simulink model "undirect_graph_disturbance_first_order_switch"  (R2020a)
settings: Solver=FixedStepAuto  StartTime=0.0  StopTime=10.0  FixedStep=0.0001  RelTol=1e-3
libraries: simulink x10, fod x1
settings Model: Creator=WangQipeng  LastModifiedBy=WangQipeng

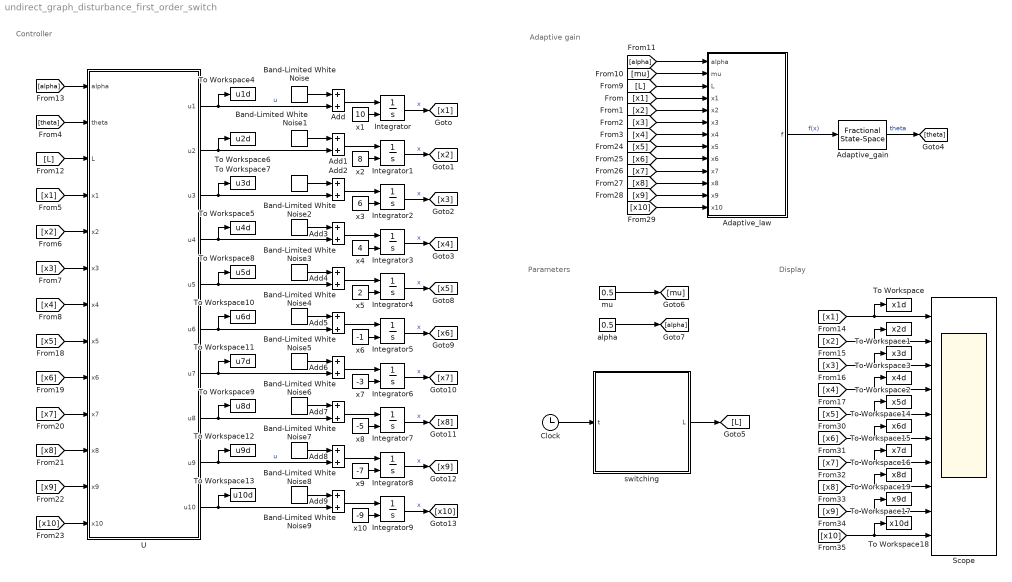
== system undirect_graph_disturbance_first_order_switch ==
  note: Controller
  note: Adaptive gain
  note: Display
  note: Parameters
  Adaptive_gain : fod/Fractional State-Space  A=0  B=1  C=1  D=0  q=0.5  iniOff=[0]  freqRange=[0.0001 10000]  approxNum=5  useRef=off  mask(FOSS){}
      settings: SourceProductName=FOMCON Toolbox
      mask Display: disp(['D^\beta \theta=f(x)'], 'TeXMode', 'On');
  Adaptive_law : MATLAB Function  TreatAsAtomicUnit=on
  Add{,1..9} (10 alike) : Sum
  Band-Limited White Noise : simulink/Sources/Band-Limited White Noise  Cov=[0.01]  Ts=0.01  seed=[23341]
  Band-Limited White Noise1 : simulink/Sources/Band-Limited White Noise  Cov=[0.01]  Ts=0.01  seed=[22141]
  Band-Limited White Noise2 : simulink/Sources/Band-Limited White Noise  Cov=[0.01]  Ts=0.01  seed=[27541]
  Band-Limited White Noise3 : simulink/Sources/Band-Limited White Noise  Cov=[0.01]  Ts=0.01  seed=[23841]
  Band-Limited White Noise4 : simulink/Sources/Band-Limited White Noise  Cov=[0.01]  Ts=0.01  seed=[25341]
  Band-Limited White Noise5 : simulink/Sources/Band-Limited White Noise  Cov=[0.01]  Ts=0.01  seed=[23261]
  Band-Limited White Noise6 : simulink/Sources/Band-Limited White Noise  Cov=[0.01]  Ts=0.01  seed=[21241]
  Band-Limited White Noise7 : simulink/Sources/Band-Limited White Noise  Cov=[0.01]  Ts=0.01  seed=[27841]
  Band-Limited White Noise8 : simulink/Sources/Band-Limited White Noise  Cov=[0.01]  Ts=0.01  seed=[23361]
  Band-Limited White Noise9 : simulink/Sources/Band-Limited White Noise  Cov=[0.01]  Ts=0.01  seed=[23521]
  Clock : Clock
  Integrator{,1..9} (10 alike) : Integrator  InitialConditionSource=external  InitialCondition=1
  Scope : Scope  NumInputPorts=10
  To Workspace : ToWorkspace  VariableName=x1d  SaveFormat=Timeseries  SampleTime=-1
  To Workspace1 : ToWorkspace  VariableName=x2d  SaveFormat=Timeseries  SampleTime=-1
  To Workspace10 : ToWorkspace  VariableName=u6d  SaveFormat=Timeseries  SampleTime=-1
  To Workspace11 : ToWorkspace  VariableName=u7d  SaveFormat=Timeseries  SampleTime=-1
  To Workspace12 : ToWorkspace  VariableName=u9d  SaveFormat=Timeseries  SampleTime=-1
  To Workspace13 : ToWorkspace  VariableName=u10d  SaveFormat=Timeseries  SampleTime=-1
  To Workspace14 : ToWorkspace  VariableName=x5d  SaveFormat=Timeseries  SampleTime=-1
  To Workspace15 : ToWorkspace  VariableName=x6d  SaveFormat=Timeseries  SampleTime=-1
  To Workspace16 : ToWorkspace  VariableName=x7d  SaveFormat=Timeseries  SampleTime=-1
  To Workspace17 : ToWorkspace  VariableName=x9d  SaveFormat=Timeseries  SampleTime=-1
  To Workspace18 : ToWorkspace  VariableName=x10d  SaveFormat=Timeseries  SampleTime=-1
  To Workspace19 : ToWorkspace  VariableName=x8d  SaveFormat=Timeseries  SampleTime=-1
  To Workspace2 : ToWorkspace  VariableName=x4d  SaveFormat=Timeseries  SampleTime=-1
  To Workspace3 : ToWorkspace  VariableName=x3d  SaveFormat=Timeseries  SampleTime=-1
  To Workspace4 : ToWorkspace  VariableName=u1d  SaveFormat=Timeseries  SampleTime=-1
  To Workspace5 : ToWorkspace  VariableName=u4d  SaveFormat=Timeseries  SampleTime=-1
  To Workspace6 : ToWorkspace  VariableName=u2d  SaveFormat=Timeseries  SampleTime=-1
  To Workspace7 : ToWorkspace  VariableName=u3d  SaveFormat=Timeseries  SampleTime=-1
  To Workspace8 : ToWorkspace  VariableName=u5d  SaveFormat=Timeseries  SampleTime=-1
  To Workspace9 : ToWorkspace  VariableName=u8d  SaveFormat=Timeseries  SampleTime=-1
  U : MATLAB Function  TreatAsAtomicUnit=on
  alpha : Constant  Value=0.5
  mu : Constant  Value=0.5
  switching : MATLAB Function  TreatAsAtomicUnit=on
  x1 : Constant  Value=10
  x10 : Constant  Value=-9
  x2 : Constant  Value=8
  x3 : Constant  Value=6
  x4 : Constant  Value=4
  x5 : Constant  Value=2
  x6 : Constant  Value=-1
  x7 : Constant  Value=-3
  x8 : Constant  Value=-5
  x9 : Constant  Value=-7
  wires:
  U/1(u1) -> To Workspace4/1, Add/2  "u"
  Adaptive_law/1(f) -> Adaptive_gain/1  "f(x)"
  U/4(u4) -> To Workspace5/1, Add3/2
  Integrator/1 -> [x1]  "x"
  [x1] -> Adaptive_law/4(x1)
  Integrator1/1 -> [x2]  "x"
  Integrator2/1 -> [x3]  "x"
  Integrator3/1 -> [x4]  "x"
  [x2] -> Adaptive_law/5(x2)
  [x3] -> Adaptive_law/6(x3)
  [x4] -> Adaptive_law/7(x4)
  Adaptive_gain/1 -> [theta]  "theta"
  [theta] -> U/2(theta)
  [x3] -> U/6(x3)
  [x4] -> U/7(x4)
  [x1] -> U/4(x1)
  [x2] -> U/5(x2)
  [L] -> Adaptive_law/3(L)
  mu/1 -> [mu]
  alpha/1 -> [alpha]
  [mu] -> Adaptive_law/2(mu)
  [alpha] -> Adaptive_law/1(alpha)
  [L] -> U/3(L)
  [alpha] -> U/1(alpha)
  x1/1 -> Integrator/2
  x2/1 -> Integrator1/2
  x3/1 -> Integrator2/2
  x4/1 -> Integrator3/2
  [x1] -> To Workspace/1, Scope/1
  [x2] -> To Workspace1/1, Scope/2
  [x3] -> To Workspace3/1, Scope/3
  [x4] -> To Workspace2/1, Scope/4
  Band-Limited White Noise/1 -> Add/1
  Add/1 -> Integrator/1
  Band-Limited White Noise1/1 -> Add1/1
  Add1/1 -> Integrator1/1
  Band-Limited White Noise2/1 -> Add2/1
  Add2/1 -> Integrator2/1
  Add3/1 -> Integrator3/1
  Band-Limited White Noise3/1 -> Add3/1
  U/3(u3) -> To Workspace7/1, Add2/2
  U/2(u2) -> To Workspace6/1, Add1/2
  U/7(u7) -> To Workspace11/1, Add6/2
  Add7/1 -> Integrator7/1
  x7/1 -> Integrator6/2
  Band-Limited White Noise5/1 -> Add5/1
  Integrator7/1 -> [x8]  "x"
  x6/1 -> Integrator5/2
  x8/1 -> Integrator7/2
  Add6/1 -> Integrator6/1
  Add5/1 -> Integrator5/1
  Add4/1 -> Integrator4/1
  U/5(u5) -> To Workspace8/1, Add4/2
  x5/1 -> Integrator4/2
  Band-Limited White Noise7/1 -> Add7/1
  Integrator4/1 -> [x5]  "x"
  Integrator6/1 -> [x7]  "x"
  Band-Limited White Noise6/1 -> Add6/1
  U/8(u8) -> To Workspace9/1, Add7/2
  Integrator5/1 -> [x6]  "x"
  U/6(u6) -> To Workspace10/1, Add5/2
  Band-Limited White Noise4/1 -> Add4/1
  Band-Limited White Noise9/1 -> Add9/1
  x10/1 -> Integrator9/2
  Add9/1 -> Integrator9/1
  U/9(u9) -> To Workspace12/1, Add8/2  "u"
  Add8/1 -> Integrator8/1
  x9/1 -> Integrator8/2
  Integrator8/1 -> [x9]  "x"
  Integrator9/1 -> [x10]  "x"
  U/10(u10) -> To Workspace13/1, Add9/2
  Band-Limited White Noise8/1 -> Add8/1
  [x10] -> U/13(x10)
  [x9] -> U/12(x9)
  [x8] -> U/11(x8)
  [x7] -> U/10(x7)
  [x6] -> U/9(x6)
  [x5] -> U/8(x5)
  [x10] -> Adaptive_law/13(x10)
  [x9] -> Adaptive_law/12(x9)
  [x8] -> Adaptive_law/11(x8)
  [x7] -> Adaptive_law/10(x7)
  [x6] -> Adaptive_law/9(x6)
  [x5] -> Adaptive_law/8(x5)
  [x6] -> To Workspace15/1, Scope/6
  [x7] -> To Workspace16/1, Scope/7
  [x8] -> To Workspace19/1, Scope/8
  [x5] -> To Workspace14/1, Scope/5
  [x10] -> To Workspace18/1, Scope/10
  [x9] -> To Workspace17/1, Scope/9
  switching/1(L) -> [L]
  Clock/1 -> switching/1(t)

== matlab function undirect_graph_disturbance_first_order_switch/U ==
  data: alpha input; u1 output; theta input; L input; x1 input; x2 input; x3 input; x4 input; u2 output; u3 output; u4 output; x5 input; x6 input; x7 input; x8 input; x9 input; x10 input; u5 output; u6 output; u7 output; u8 output; u9 output; u10 output
function [u1,u2,u3,u4,u5,u6,u7,u8,u9,u10] = protocol(alpha,theta,L,x1,x2,x3,x4,x5,x6,x7,x8,x9,x10)
x = [x1;x2;x3;x4;x5;x6;x7;x8;x9;x10];
temp = L * x;
temp_u1 = temp(1);
temp_u2 = temp(2);
temp_u3 = temp(3);
temp_u4 = temp(4);
temp_u5 = temp(5);
temp_u6 = temp(6);
temp_u7 = temp(7);
temp_u8 = temp(8);
temp_u9 = temp(9);
temp_u10 = temp(10);


u1 = -theta * sign(temp_u1) * abs(temp_u1)^(1-alpha);
u2 = -theta * sign(temp_u2) * abs(temp_u2)^(1-alpha);
u3 = -theta * sign(temp_u3) * abs(temp_u3)^(1-alpha);
u4 = -theta * sign(temp_u4) * abs(temp_u4)^(1-alpha);
u5 = -theta * sign(temp_u5) * abs(temp_u5)^(1-alpha);
u6 = -theta * sign(temp_u6) * abs(temp_u6)^(1-alpha);
u7 = -theta * sign(temp_u7) * abs(temp_u7)^(1-alpha);
u8 = -theta * sign(temp_u8) * abs(temp_u8)^(1-alpha);
u9 = -theta * sign(temp_u9) * abs(temp_u9)^(1-alpha);
u10 = -theta * sign(temp_u10) * abs(temp_u10)^(1-alpha);

== matlab function undirect_graph_disturbance_first_order_switch/Adaptive_law ==
  data: alpha input; f output; mu input; L input; x1 input; x2 input; x3 input; x4 input; x5 input; x6 input; x7 input; x8 input; x9 input; x10 input
function f = Lyapunov_Like(alpha,mu,L,x1,x2,x3,x4,x5,x6,x7,x8,x9,x10)
x = [x1;x2;x3;x4;x5;x6;x7;x8;x9;x10];
P_L = 2 * x' * L * x;
f = mu * abs(P_L)^(alpha/2);

== matlab function undirect_graph_disturbance_first_order_switch/switching ==
  data: t input; L output
function L = Switch(t)
if t<1
    L = [2 -1 0 0 0 0 0 0 0 -1;
 -1 2 -1 0 0 0 0 0 0 0;
 0 -1 2 -1 0 0 0 0 0 0;
 0 0 -1 2 -1 0 0 0 0 0;
 0 0 0 -1 2 -1 0 0 0 0;
 0 0 0 0 -1 2 -1 0 0 0;
 0 0 0 0 0 -1 2 -1 0 0;
 0 0 0 0 0 0 -1 2 -1 0;
 0 0 0 0 0 0 0 -1 2 -1;
 -1 0 0 0 0 0 0 0 -1 2];
elseif t<6
    L = [3 0 0 -1 0 -1 0 -1 0 0;
 0 3 0 0 -1 0 -1 0 -1 0;
 0 0 3 0 0 -1 0 -1 0 -1;
 -1 0 0 3 0 0 -1 0 -1 0;
 0 -1 0 0 3 0 0 -1 0 -1;
 -1 0 -1 0 0 3 0 0 -1 0;
 0 -1 0 -1 0 0 3 0 0 -1;
 -1 0 -1 0 -1 0 0 3 0 0;
 0 -1 0 -1 0 -1 0 0 3 0;
 0 0 -1 0 -1 0 -1 0 0 3];
else
    L = [2 -1 0 0 0 0 0 0 0 -1;
 -1 2 -1 0 0 0 0 0 0 0;
 0 -1 2 -1 0 0 0 0 0 0;
 0 0 -1 2 -1 0 0 0 0 0;
 0 0 0 -1 2 -1 0 0 0 0;
 0 0 0 0 -1 2 -1 0 0 0;
 0 0 0 0 0 -1 2 -1 0 0;
 0 0 0 0 0 0 -1 2 -1 0;
 0 0 0 0 0 0 0 -1 2 -1;
 -1 0 0 0 0 0 0 0 -1 2];
end
